simulink model "sampleModel205"  (R2021b)
settings: Solver=VariableStepAuto  StartTime=0.0  StopTime=10.0  RelTol=1e-3
undefined symbols (not defined in the file or in its folder): Newton, Raphson
libraries: simulink x5, slpidlib x2
settings Model: Creator=user  LastModifiedBy=user

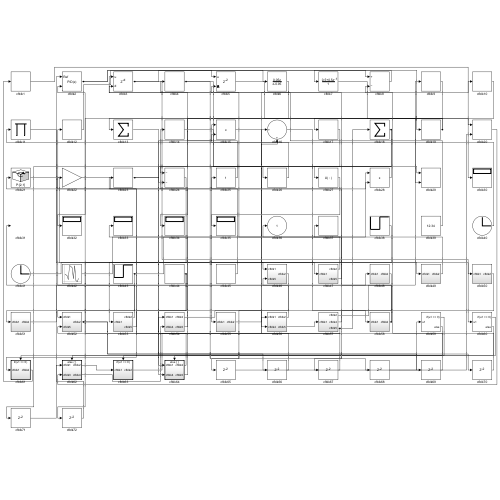
[thumbnail: Simulink's stored preview of the top-level diagram]
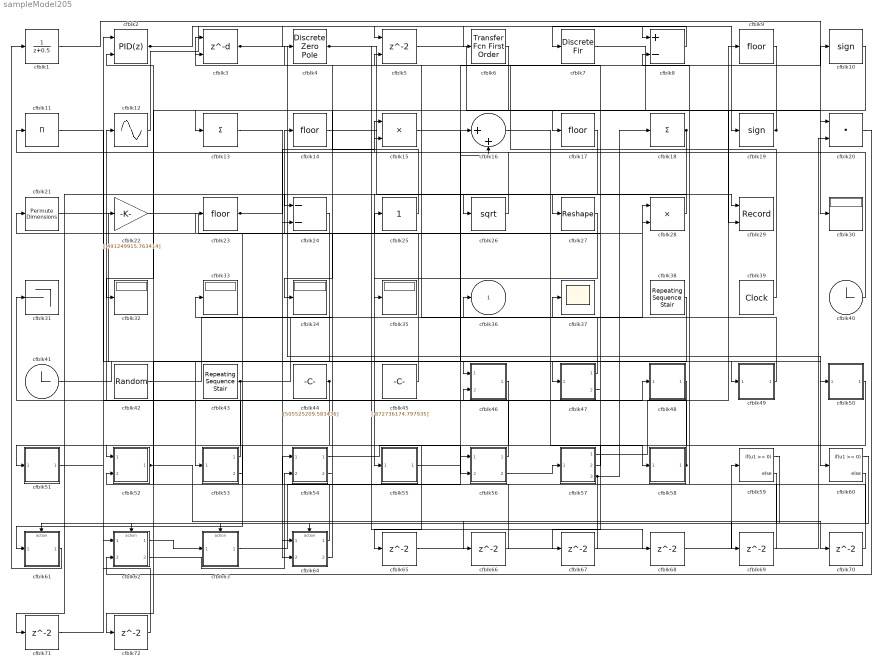
== system sampleModel205 ==
  cfblk1 : DiscreteTransferFcn  SampleTime=1
  cfblk10 : Signum
  cfblk11 : Product  Inputs=*
  cfblk12 : Sin  TimeSource=Use external signal  SampleTime=0
  cfblk13 : Sum  Inputs=+
  cfblk{9,14,17,23} (4 alike) : Rounding
  cfblk15 : Product
  cfblk16 : Sum  Inputs=|++
  cfblk18 : Sum  Inputs=+
  cfblk19 : Signum
  cfblk2 : slpidlib/PID Controller (2DOF)  Controller=PID  Form=Parallel  TimeDomain=Discrete-time  UseExternalTs=off  SampleTime=1  IntegratorMethod=Forward Euler  FilterMethod=Forward Euler  ControllerParametersSource=internal  P=1  I=1  D=0  UseFilter=on  N=100  b=1  c=1  TunerSelectOption=Transfer Function Based (PID Tuner App)  InitialConditionSource=internal  InitialConditionForIntegrator=0  InitialConditionForFilter=0  DifferentiatorICPrevScaledInput=0  ExternalReset=none  TrackingMode=off  Kt=1  LimitOutput=off  SatLimitsSource=internal  UpperSaturationLimit=inf  LowerSaturationLimit=-inf  LinearizeAsGain=off  AntiWindupMode=none  Kb=1  POutMin=[]  POutMax=[]  IOutMin=[]  IOutMax=[]  DOutMin=[]  DOutMax=[]  NOutMin=[]  NOutMax=[]  bOutMin=[]  bOutMax=[]  cOutMin=[]  cOutMax=[]  SumOutMin=[]  SumOutMax=[]  SaturationOutMin=[]  SaturationOutMax=[]  PParamMin=[]  PParamMax=[]  IParamMin=[]  IParamMax=[]  DParamMin=[]  DParamMax=[]  NParamMin=[]  NParamMax=[]  bParamMin=[]  bParamMax=[]  cParamMin=[]  cParamMax=[]  KbParamMin=[]  KbParamMax=[]  KtParamMin=[]  KtParamMax=[]  KbOutMin=[]  KbOutMax=[]  KtOutMin=[]  KtOutMax=[]  IntegratorOutMin=[]  IntegratorOutMax=[]  FilterOutMin=[]  FilterOutMax=[]  SumI1OutMin=[]  SumI1OutMax=[]  SumI2OutMin=[]  SumI2OutMax=[]  SumI3OutMin=[]  SumI3OutMax=[]  SumI4OutMin=[]  SumI4OutMax=[]  SumDOutMin=[]  SumDOutMax=[]  Sum1OutMin=[]  Sum1OutMax=[]  Sum2OutMin=[]  Sum2OutMax=[]  Sum3OutMin=[]  Sum3OutMax=[]  DifferentiatorOutMin=[]  DifferentiatorOutMax=[]  FilterDiffOutCoefMin=[]  FilterDiffOutCoefMax=[]  ReciprocalOutMin=[]  ReciprocalOutMax=[]  SumDenOutMin=[]  SumDenOutMax=[]  SumNumOutMin=[]  SumNumOutMax=[]  DivideOutMin=[]  DivideOutMax=[]  UdiffTsProdOutMin=[]  UdiffTsProdOutMax=[]  NTsProdOutMin=[]  NTsProdOutMax=[]  UintegralTsProdOutMin=[]  UintegralTsProdOutMax=[]  UngainTsProdOutMin=[]  UngainTsProdOutMax=[]  IntegratorContinuousStateAttributes=''  IntegratorStateMustResolveToSignalObject=off  IntegratorRTWStateStorageClass=Auto  FilterContinuousStateAttributes=''  FilterStateMustResolveToSignalObject=off  FilterRTWStateStorageClass=Auto  ParallelPVariant=InternalParameters  IdealPVariant=Disabled  IVariant=InternalParameters  DVariant=InternalParameters  bVariant=InternalParameters  cVariant=InternalParameters  IntegratorVariant=Discrete  SatVariant=Disabled  AWVariant=Passthrough  PCopyVariant=Disabled  TRVariant=Disabled  FdbkBlocksVariant=Forward  IdealPFdbkVariant=Disabled  SatFdbkVariant=Disabled  DerivativeFilterVariant=ForwardEulerFilter  NVariant=InternalParameters  NCopyVariant=Disabled  FilterICVariant=InternalICsFilter  IntegratorICVariant=InternalICs  ExternalResetVariant=Disabled  TRSumVariant=Passthrough  SumFdbkVariant=Disabled  SumVariant=Sum_PID  TsampFilterVariant=InternalTs  TsampNgainVariant=Passthrough  TsampIntegralVariant=Passthrough  ExternalSaturationOutDataTypeStr=Inherit: Same as second input
      settings: SourceProductBaseCode=SL
  cfblk20 : DotProduct  InputSameDT=on  OutDataTypeStr=Inherit: Inherit via internal rule
  cfblk21 : PermuteDimensions
  cfblk22 : Gain  Gain=[-491249915.763414]
  cfblk24 : Sum  Inputs=--
  cfblk25 : simulink/Math Operations/Slider Gain  gain=1  low=0  high=2
  cfblk26 : Sqrt  SaturateOnIntegerOverflow=on
  cfblk27 : Reshape
  cfblk28 : Product  Inputs=**
  cfblk29 : Record  FileSettingsInternal="{\"entries\":[{\"content\":{\"excelSettings\":{\"content\":{},\"type\":\"Streamout.ExcelSettings\"}},\"type\":\"Streamout.FileSettingStorage\",\"uuid\":\"f730e0e7-53fe-464a-9a82-0900e3942749\"}],\"packageUris\":[\"http://schema.mathworks.com/mf0/streamout_blocks/R2020a\"],\"version\":\"1.0\"}"  Layout=[1 1]  SignalsInternal="{\"entries\":[{\"content\":{\"signals\":[{\"content\":{\"blockPath\":[\"sampleModel205/cfblk29\"],\"channel\":[],\"dimensions\":[1,1],\"domain\":\"sampleModel205/cfblk29\",\"lineColor\":\"#a2142f\",\"plots\":[1],\"port\":1,\"sid\":[\"\"],\"signalID\":7899,\"signalName\":\"cfblk4\"},\"type\":\"RecordBlkView.Signal\",\"uuid\":\"9c209e98-6881-4a35-a685-ad8e26a1ce75\"},{\"content\":{\"blockPath\":[\"sampleModel205/cfblk29\"],\"channel\":[],\"dimensions\":[1],\"domain\":\"sampleModel205/cfblk29\",\"lineColor\":\"#139fff\",\"plots\":[1],\"port\":2,\"sid\":[\"\"],\"signalID\":7903,\"signalName\":\"cfblk5\"},\"type\":\"RecordBlkView.Signal\",\"uuid\":\"49d15c18-b6c9-4e42-b01f-ba5386945ad3\"}]},\"type\":\"RecordBlkView.InputSignals\",\"uuid\":\"0b933341-382b-4c1e-8b63-004dbd7fd521\"}],\"packageUris\":[\"http://schema.mathworks.com/mf0/streamout_blocks/R2020a\"],\"version\":\"1.0\"}"  VisualizationBindings="{\"xyplotplugin\":{\"info\":[{\"series\":[{\"bindingParametersList\":[{\"parameter\":\"X-Axis\",\"signalID\":7899,\"signalName\":\"cfblk4\"},{\"parameter\":\"Y-Axis\",\"signalID\":7903,\"signalName\":\"cfblk5\"}],\"seriesID\":36192}],\"subplotID\":1}]}}"  CompatibilityTag=XY
  cfblk3 : Delay  DelayLengthSource=Input port  SampleTime=1
      settings: InputPortMap=u0,p1
  cfblk{30,32..35} (5 alike) : Display
  cfblk31 : Terminator
  cfblk37 : Scope
  cfblk38 : simulink/Sources/Repeating Sequence Stair  OutValues=[-948918117.182882, -63589175.997918]  tsamp=-1  OutMin=[]  OutMax=[]  OutDataTypeStr=double  OutputDataTypeScalingMode=double  OutDataType=fixdt(0,8)  ConRadixGroup=Best Precision: Vector-wise  OutScaling=2^-12
  cfblk39 : DigitalClock
  cfblk4 : DiscreteZeroPole  Poles=[0 0.5]  Gain=1
  cfblk40 : Clock
  cfblk41 : Clock
  cfblk42 : RandomNumber  Mean=[64196.223504]  Variance=[2477.301386]  Seed=[337225866.000000]  SampleTime=0.1
  cfblk43 : simulink/Sources/Repeating Sequence Stair  OutValues=[924954321.616893, 939022087.631474]  tsamp=-1  OutMin=[]  OutMax=[]  OutDataTypeStr=double  OutputDataTypeScalingMode=double  OutDataType=fixdt(0,8)  ConRadixGroup=Best Precision: Vector-wise  OutScaling=2^-12
  cfblk44 : Constant  Value=[505525209.583436]  SampleTime=1
  cfblk45 : Constant  Value=[-872736174.797935]  SampleTime=1
  cfblk46 : Subsystem
  cfblk47 : Subsystem
  cfblk48 : Subsystem
  cfblk49 : Subsystem
  cfblk5 : Delay  ShowEnablePort=on  SampleTime=1
      settings: InputPortMap=u0,e6
  cfblk50 : Subsystem
  cfblk51 : Subsystem
  cfblk52 : Subsystem
  cfblk53 : Subsystem
  cfblk54 : Subsystem
  cfblk55 : Subsystem
  cfblk56 : Subsystem
  cfblk57 : Subsystem
  cfblk58 : Subsystem
  cfblk59 : If  IfExpression=u1 >= 0  SampleTime=1
  cfblk6 : simulink/Discrete/Transfer Fcn First Order  PoleZ=0.95  ICPrevOutput=0.0  DoSatur=off
  cfblk60 : If  IfExpression=u1 >= 0  SampleTime=1
  cfblk61 : Subsystem  TreatAsAtomicUnit=on
  cfblk62 : Subsystem  TreatAsAtomicUnit=on
  cfblk63 : Subsystem  TreatAsAtomicUnit=on
  cfblk64 : Subsystem  TreatAsAtomicUnit=on
  cfblk{65..72} (8 alike) : Delay  SampleTime=1
  cfblk7 : DiscreteFir  SampleTime=1
  cfblk8 : Sum  Inputs=+-
  cfblk36 : Outport
  wires:
  cfblk21/1 -> cfblk47/1(cfblk1)
  cfblk53/1(cfblk2) -> cfblk12/1
  cfblk3/1 -> cfblk60/1, cfblk6/1
  cfblk45/1 -> cfblk14/1
  cfblk44/1 -> cfblk61/1(cfblk1), cfblk64/2(cfblk4)
  cfblk62/1(cfblk2) -> cfblk63/1(cfblk1)
  cfblk6/1 -> cfblk32/1
  cfblk12/1 -> cfblk19/1
  cfblk58/1(cfblk2) -> cfblk37/1, cfblk46/2(cfblk5)
  cfblk18/1 -> cfblk24/2, cfblk71/1
  cfblk9/1 -> cfblk34/1
  cfblk1/1 -> cfblk30/1
  cfblk48/1(cfblk2) -> cfblk52/1(cfblk1)
  cfblk25/1 -> cfblk4/1
  cfblk17/1 -> cfblk55/1(cfblk1)
  cfblk23/1 -> cfblk15/2, cfblk66/1
  cfblk57/1(cfblk2) -> cfblk9/1
  cfblk11/1 -> cfblk46/1(cfblk1)
  cfblk47/1(cfblk2) -> cfblk36/1
  cfblk14/1 -> cfblk26/1
  cfblk10/1 -> cfblk24/1
  cfblk52/1(cfblk2) -> cfblk69/1, cfblk70/1
  cfblk27/1 -> cfblk35/1
  cfblk19/1 -> cfblk17/1, cfblk13/1
  cfblk43/1 -> cfblk51/1(cfblk1), cfblk16/2
  cfblk62/2(cfblk4) -> cfblk54/2(cfblk4)
  cfblk8/1 -> cfblk7/1
  cfblk55/1(cfblk2) -> cfblk10/1
  cfblk61/1(cfblk2) -> cfblk1/1
  cfblk4/1 -> cfblk29/1, cfblk68/1
  cfblk63/1(cfblk2) -> cfblk16/1
  cfblk39/1 -> cfblk3/1
  cfblk51/1(cfblk2) -> cfblk48/1(cfblk1)
  cfblk57/2(cfblk4) -> cfblk3/2
  cfblk5/1 -> cfblk29/2
  cfblk2/1 -> cfblk5/1, cfblk8/1
  cfblk56/1(cfblk2) -> cfblk31/1
  cfblk47/2(cfblk5) -> cfblk25/1
  cfblk16/1 -> cfblk58/1(cfblk1)
  cfblk42/1 -> cfblk28/1
  cfblk41/1 -> cfblk49/1(cfblk1)
  cfblk15/1 -> cfblk50/1(cfblk1)
  cfblk13/1 -> cfblk64/1(cfblk1)
  cfblk40/1 -> cfblk11/1
  cfblk53/2(cfblk5) -> cfblk22/1
  cfblk7/1 -> cfblk20/1
  cfblk22/1 -> cfblk28/2
  cfblk28/1 -> cfblk27/1
  cfblk20/1 -> cfblk62/2(cfblk3)
  cfblk26/1 -> cfblk15/1
  cfblk38/1 -> cfblk53/1(cfblk1)
  cfblk57/3(cfblk5) -> cfblk52/2(cfblk5), cfblk18/1
  cfblk49/1(cfblk2) -> cfblk5/2
  cfblk56/2(cfblk5) -> cfblk57/1(cfblk1)
  cfblk64/1(cfblk2) -> cfblk23/1
  cfblk54/1(cfblk2) -> cfblk56/2(cfblk4)
  cfblk64/2(cfblk5) -> cfblk21/1
  cfblk54/2(cfblk5) -> cfblk33/1
  cfblk59/1 -> cfblk61/Action
  cfblk59/2 -> cfblk62/Action
  cfblk60/1 -> cfblk63/Action
  cfblk60/2 -> cfblk64/Action
  cfblk46/1(cfblk2) -> cfblk65/1
  cfblk65/1 -> cfblk59/1
  cfblk66/1 -> cfblk2/2
  cfblk50/1(cfblk2) -> cfblk67/1
  cfblk67/1 -> cfblk56/1(cfblk1)
  cfblk68/1 -> cfblk20/2
  cfblk69/1 -> cfblk54/1(cfblk1)
  cfblk70/1 -> cfblk8/2
  cfblk71/1 -> cfblk2/1
  cfblk24/1 -> cfblk72/1
  cfblk72/1 -> cfblk62/1(cfblk1)

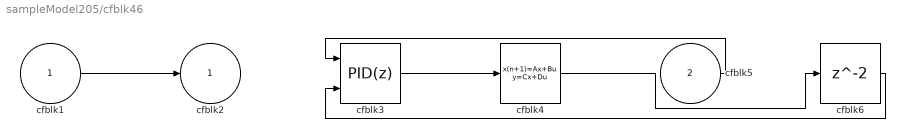
== system sampleModel205/cfblk46 ==
  cfblk1 : Inport
  cfblk5 : Inport  Port=2
  cfblk3 : slpidlib/PID Controller (2DOF)  Controller=PID  Form=Parallel  TimeDomain=Discrete-time  UseExternalTs=off  SampleTime=1  IntegratorMethod=Forward Euler  FilterMethod=Forward Euler  ControllerParametersSource=internal  P=1  I=1  D=0  UseFilter=on  N=100  b=1  c=1  TunerSelectOption=Transfer Function Based (PID Tuner App)  InitialConditionSource=internal  InitialConditionForIntegrator=0  InitialConditionForFilter=0  DifferentiatorICPrevScaledInput=0  ExternalReset=none  TrackingMode=off  Kt=1  LimitOutput=off  SatLimitsSource=internal  UpperSaturationLimit=inf  LowerSaturationLimit=-inf  LinearizeAsGain=off  AntiWindupMode=none  Kb=1  POutMin=[]  POutMax=[]  IOutMin=[]  IOutMax=[]  DOutMin=[]  DOutMax=[]  NOutMin=[]  NOutMax=[]  bOutMin=[]  bOutMax=[]  cOutMin=[]  cOutMax=[]  SumOutMin=[]  SumOutMax=[]  SaturationOutMin=[]  SaturationOutMax=[]  PParamMin=[]  PParamMax=[]  IParamMin=[]  IParamMax=[]  DParamMin=[]  DParamMax=[]  NParamMin=[]  NParamMax=[]  bParamMin=[]  bParamMax=[]  cParamMin=[]  cParamMax=[]  KbParamMin=[]  KbParamMax=[]  KtParamMin=[]  KtParamMax=[]  KbOutMin=[]  KbOutMax=[]  KtOutMin=[]  KtOutMax=[]  IntegratorOutMin=[]  IntegratorOutMax=[]  FilterOutMin=[]  FilterOutMax=[]  SumI1OutMin=[]  SumI1OutMax=[]  SumI2OutMin=[]  SumI2OutMax=[]  SumI3OutMin=[]  SumI3OutMax=[]  SumI4OutMin=[]  SumI4OutMax=[]  SumDOutMin=[]  SumDOutMax=[]  Sum1OutMin=[]  Sum1OutMax=[]  Sum2OutMin=[]  Sum2OutMax=[]  Sum3OutMin=[]  Sum3OutMax=[]  DifferentiatorOutMin=[]  DifferentiatorOutMax=[]  FilterDiffOutCoefMin=[]  FilterDiffOutCoefMax=[]  ReciprocalOutMin=[]  ReciprocalOutMax=[]  SumDenOutMin=[]  SumDenOutMax=[]  SumNumOutMin=[]  SumNumOutMax=[]  DivideOutMin=[]  DivideOutMax=[]  UdiffTsProdOutMin=[]  UdiffTsProdOutMax=[]  NTsProdOutMin=[]  NTsProdOutMax=[]  UintegralTsProdOutMin=[]  UintegralTsProdOutMax=[]  UngainTsProdOutMin=[]  UngainTsProdOutMax=[]  IntegratorContinuousStateAttributes=''  IntegratorStateMustResolveToSignalObject=off  IntegratorRTWStateStorageClass=Auto  FilterContinuousStateAttributes=''  FilterStateMustResolveToSignalObject=off  FilterRTWStateStorageClass=Auto  ParallelPVariant=InternalParameters  IdealPVariant=Disabled  IVariant=InternalParameters  DVariant=InternalParameters  bVariant=InternalParameters  cVariant=InternalParameters  IntegratorVariant=Discrete  SatVariant=Disabled  AWVariant=Passthrough  PCopyVariant=Disabled  TRVariant=Disabled  FdbkBlocksVariant=Forward  IdealPFdbkVariant=Disabled  SatFdbkVariant=Disabled  DerivativeFilterVariant=ForwardEulerFilter  NVariant=InternalParameters  NCopyVariant=Disabled  FilterICVariant=InternalICsFilter  IntegratorICVariant=InternalICs  ExternalResetVariant=Disabled  TRSumVariant=Passthrough  SumFdbkVariant=Disabled  SumVariant=Sum_PID  TsampFilterVariant=InternalTs  TsampNgainVariant=Passthrough  TsampIntegralVariant=Passthrough  ExternalSaturationOutDataTypeStr=Inherit: Same as second input
      settings: SourceProductBaseCode=SL
  cfblk4 : DiscreteStateSpace
  cfblk6 : Delay  SampleTime=1
  cfblk2 : Outport
  wires:
  cfblk5/1 -> cfblk3/1
  cfblk3/1 -> cfblk4/1
  cfblk1/1 -> cfblk2/1
  cfblk4/1 -> cfblk6/1
  cfblk6/1 -> cfblk3/2

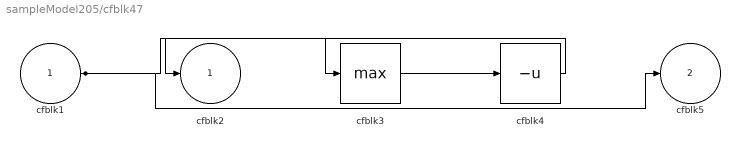
== system sampleModel205/cfblk47 ==
  cfblk1 : Inport
  cfblk3 : MinMax  Function=max
  cfblk4 : UnaryMinus
  cfblk2 : Outport
  cfblk5 : Outport  Port=2
  wires:
  cfblk4/1 -> cfblk2/1
  cfblk1/1 -> cfblk5/1, cfblk3/1
  cfblk3/1 -> cfblk4/1

== system sampleModel205/cfblk48 ==
  cfblk1 : Inport
  cfblk3 : DiscreteFir  SampleTime=1
  cfblk4 : Constant  Value=[895810020.108873]  SampleTime=1
  cfblk2 : Outport
  wires:
  cfblk4/1 -> cfblk2/1
  cfblk1/1 -> cfblk3/1

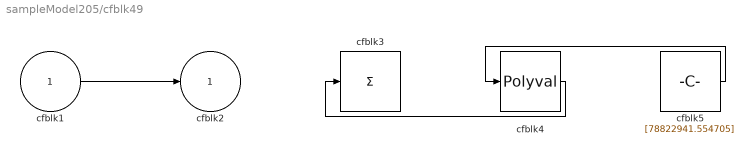
== system sampleModel205/cfblk49 ==
  cfblk1 : Inport
  cfblk3 : Sum  Inputs=+
  cfblk4 : Polyval  Coefs=[ +2.081618890e-019, -1.441693666e-014, +4.719686976e-010, -8.536869453e-006, +1.621573104e-001, -8.087801117e+001 ]
  cfblk5 : Constant  Value=[78822941.554705]  SampleTime=1
  cfblk2 : Outport
  wires:
  cfblk1/1 -> cfblk2/1
  cfblk5/1 -> cfblk4/1
  cfblk4/1 -> cfblk3/1

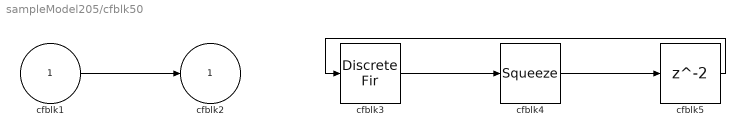
== system sampleModel205/cfblk50 ==
  cfblk1 : Inport
  cfblk3 : DiscreteFir  SampleTime=1
  cfblk4 : Squeeze
  cfblk5 : Delay  SampleTime=1
  cfblk2 : Outport
  wires:
  cfblk1/1 -> cfblk2/1
  cfblk3/1 -> cfblk4/1
  cfblk4/1 -> cfblk5/1
  cfblk5/1 -> cfblk3/1

== system sampleModel205/cfblk51 ==
  cfblk1 : Inport
  cfblk3 : DotProduct  InputSameDT=on  OutDataTypeStr=Inherit: Inherit via internal rule
  cfblk4 : UnaryMinus
  cfblk2 : Outport
  wires:
  cfblk1/1 -> cfblk3/1, cfblk4/1
  cfblk4/1 -> cfblk3/2
  cfblk3/1 -> cfblk2/1

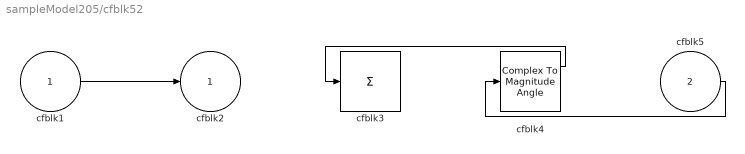
== system sampleModel205/cfblk52 ==
  cfblk1 : Inport
  cfblk5 : Inport  Port=2
  cfblk3 : Sum  Inputs=+
  cfblk4 : ComplexToMagnitudeAngle
  cfblk2 : Outport
  wires:
  cfblk4/1 -> cfblk3/1
  cfblk5/1 -> cfblk4/1
  cfblk1/1 -> cfblk2/1

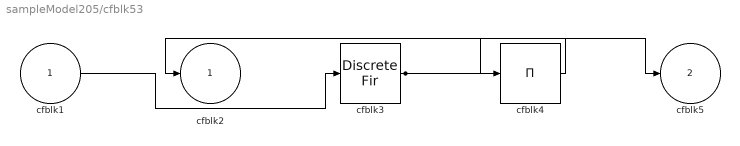
== system sampleModel205/cfblk53 ==
  cfblk1 : Inport
  cfblk3 : DiscreteFir  SampleTime=1
  cfblk4 : Product  Inputs=*
  cfblk2 : Outport
  cfblk5 : Outport  Port=2
  wires:
  cfblk3/1 -> cfblk4/1, cfblk5/1
  cfblk4/1 -> cfblk2/1
  cfblk1/1 -> cfblk3/1

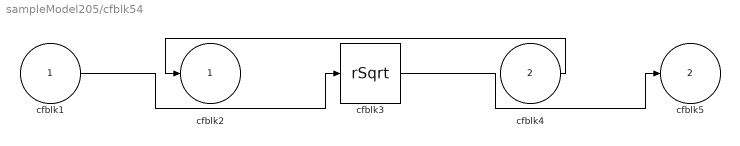
== system sampleModel205/cfblk54 ==
  cfblk1 : Inport
  cfblk4 : Inport  Port=2
  cfblk3 : Sqrt  Operator=rSqrt  AlgorithmType=Newton-Raphson  SaturateOnIntegerOverflow=on
  cfblk2 : Outport
  cfblk5 : Outport  Port=2
  wires:
  cfblk4/1 -> cfblk2/1
  cfblk1/1 -> cfblk3/1
  cfblk3/1 -> cfblk5/1

== system sampleModel205/cfblk55 ==
  cfblk1 : Inport
  cfblk3 : Sqrt  SaturateOnIntegerOverflow=on
  cfblk2 : Outport
  wires:
  cfblk1/1 -> cfblk2/1, cfblk3/1

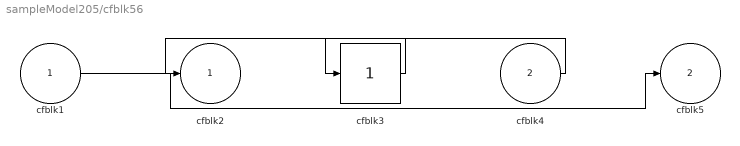
== system sampleModel205/cfblk56 ==
  cfblk1 : Inport
  cfblk4 : Inport  Port=2
  cfblk3 : simulink/Math Operations/Slider Gain  gain=1  low=0  high=2
  cfblk2 : Outport
  cfblk5 : Outport  Port=2
  wires:
  cfblk4/1 -> cfblk3/1
  cfblk1/1 -> cfblk5/1
  cfblk3/1 -> cfblk2/1

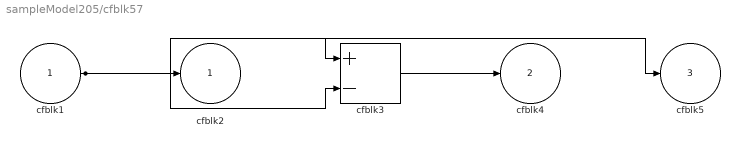
== system sampleModel205/cfblk57 ==
  cfblk1 : Inport
  cfblk3 : Sum  Inputs=+-
  cfblk2 : Outport
  cfblk4 : Outport  Port=2
  cfblk5 : Outport  Port=3
  wires:
  cfblk3/1 -> cfblk4/1
  cfblk1/1 -> cfblk3/1, cfblk5/1, cfblk3/2, cfblk2/1

== system sampleModel205/cfblk58 ==
  cfblk1 : Inport
  cfblk3 : Signum
  cfblk2 : Outport
  wires:
  cfblk1/1 -> cfblk2/1, cfblk3/1

== system sampleModel205/cfblk61 ==
  cfblk1 : Inport
  Action Port : ActionPort  ActionPortLabel=if(u1 >= 0)
  cfblk3 : DiscreteStateSpace  SampleTime=-1
  cfblk2 : Outport
  wires:
  cfblk1/1 -> cfblk2/1, cfblk3/1

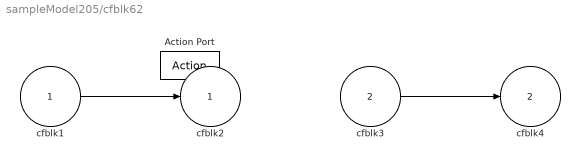
== system sampleModel205/cfblk62 ==
  cfblk1 : Inport
  cfblk3 : Inport  Port=2
  Action Port : ActionPort  ActionPortLabel=else
  cfblk2 : Outport
  cfblk4 : Outport  Port=2
  wires:
  cfblk3/1 -> cfblk4/1
  cfblk1/1 -> cfblk2/1

== system sampleModel205/cfblk63 ==
  cfblk1 : Inport
  Action Port : ActionPort  ActionPortLabel=if(u1 >= 0)
  cfblk3 : Math  SaturateOnIntegerOverflow=on
  cfblk2 : Outport
  wires:
  cfblk1/1 -> cfblk3/1
  cfblk3/1 -> cfblk2/1

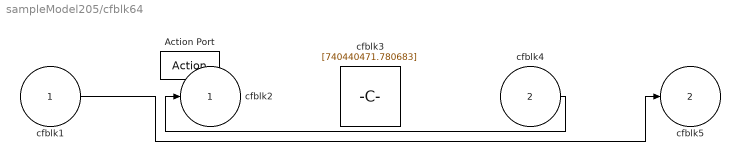
== system sampleModel205/cfblk64 ==
  cfblk1 : Inport
  cfblk4 : Inport  Port=2
  Action Port : ActionPort  ActionPortLabel=else
  cfblk3 : Constant  Value=[740440471.780683]  SampleTime=1
  cfblk2 : Outport
  cfblk5 : Outport  Port=2
  wires:
  cfblk4/1 -> cfblk2/1
  cfblk1/1 -> cfblk5/1
